simulink library "modVehicle000_cl"  (R2018b)
settings: Solver=VariableStepAuto  StartTime=0.0  StopTime=10.0  RelTol=1e-3
undefined symbols (not defined in the file): constantNormVelBool, constantVelBool, constantVelMag, env, initAngRates, Jinv, m, Minv, MMAddBool, MMOverrideBool, radialMotionBool, sixDoFDynamics, sixDoFDynamics_ul, startControl, vhcl
libraries: vrlib x3, vectorNormalizer_ul x3, eulAng2RotMat_ul x2, dragTurbine_ul x1, fluidDynamicSurface_cl x1, simulink x1, eulDot x1, tethersMoment_cl x1, thrAttachPtKinematics_ul x1
settings Model: Creator=mcobb  LastModifiedBy=mcobb

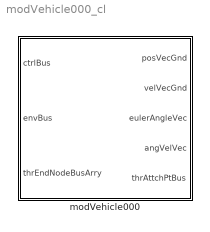
== system modVehicle000_cl ==
  modVehicle000 : Subsystem  VariantControl=VSS_vehicle_vehicle000  mask{vcl=vhcl, rho=env.water.density.Value, grav=env.gravAccel.Value}
      mask prompts: vcl "Vehicle"; rho "Fluid Density"; grav "Gravity"
      mask DialogControl Container9 Prompt: General
      mask DialogControl Container5 Prompt: Vehicle object
      mask DialogControl ParameterGroupVar Prompt: Environmental
      mask Display:
      | image('kite.jpg',[100 100 601 528]/4,'on')
      | 
      | port_label('input',1,'ctrlBus')
      | port_label('input',2,'envBus')
      | port_label('input',3,'thrEndNodeBusArry')
      | 
      | port_label('output',1,'posVecGnd')
      | port_label('output',2,'velVecGnd')
      | port_label('output',3,'eulAng')
      | port_label('output',4,'angVelVec')
      | port_label('output',5,'thrAttchPtBus')

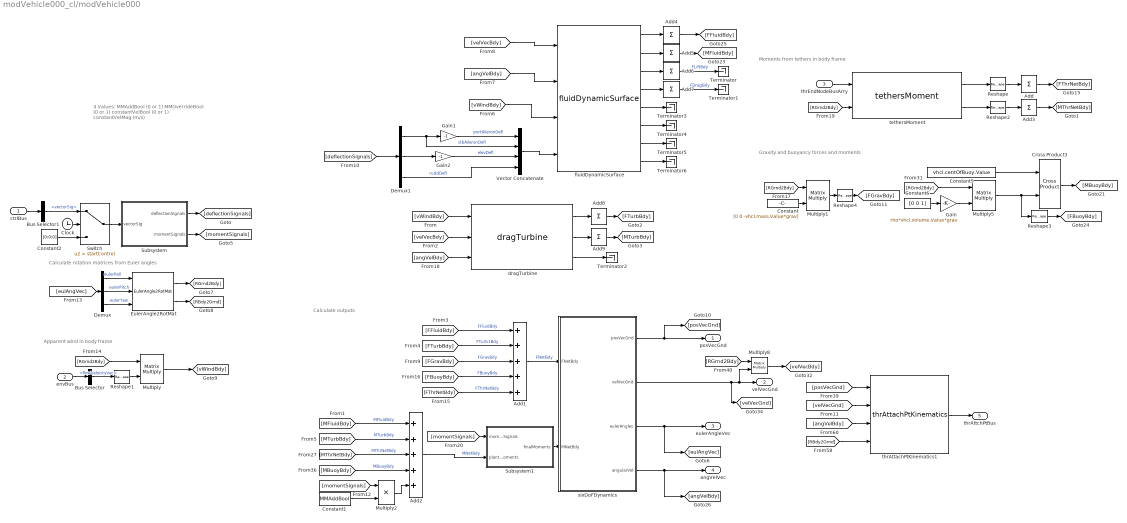
== system modVehicle000_cl/modVehicle000 ==
  note: 4 Values:
      | MMAddBool (0 or 1)
      | MMOverrideBool (0 or 1)
      | constantVelBool (0 or 1)
      | constantVelMag (m/s)
  note: Calculate outputs
  note: Apparent wind in body frame
  note: Calculate rotation matrices from Euler angles
  note: Gravity and buoyancy forces and moments
  note: Moments from tethers in body frame
  ctrlBus : Inport  OutDataTypeStr=Bus: fltCtrlBus
  envBus : Inport  Port=2  OutDataTypeStr=Bus: envBus
  thrEndNodeBusArry : Inport  Port=3
  Add : Sum  Inputs=+  CollapseMode=Specified dimension  CollapseDim=2
  Add1 : Sum  Inputs=+++++
  Add2 : Sum  Inputs=+++++
  Add3 : Sum  Inputs=+  CollapseMode=Specified dimension  CollapseDim=2
  Add{4..9} (6 alike) : Sum  Inputs=1  CollapseMode=Specified dimension  CollapseDim=2
  Bus Selector : BusSelector  OutputSignals=flowVelocityVec
  Bus Selector1 : BusSelector  OutputSignals=vectorSig
  Clock : Clock
  Constant : Constant  Value=[0 0 -vhcl.mass.Value*grav]
  Constant1 : Constant  Value=MMAddBool
  Constant2 : Constant  Value=[0;0;0]
  Constant5 : Constant  Value=vhcl.centOfBuoy.Value
  Constant6 : Constant  Value=[0 0 1]
  Cross Product3 : vrlib/Utilities/Cross Product
      settings: SourceProductBaseCode=VR
  Demux : Demux  Outputs=3
  Demux1 : Demux  Outputs=3
  EulerAngle2RotMat : eulAng2RotMat_ul/EulerAngle2RotMat  SystemSampleTime=-1
  Gain : Gain  Gain=rho*vhcl.volume.Value*grav
  Gain1 : Gain  Gain=-1
  Gain2 : Gain  Gain=-1
  Multiply{,1,5,8} (4 alike) : Product  Multiplication=Matrix(*)
  Multiply2 : Product
  Reshape : Reshape  OutputDimensionality=Customize  OutputDimensions=[3 vhcl.numTethers.Value]
  Reshape1 : Reshape  OutputDimensionality=Column vector (2-D)
  Reshape2 : Reshape  OutputDimensionality=Customize  OutputDimensions=[3 vhcl.numTethers.Value]
  Reshape3 : Reshape  OutputDimensionality=Column vector (2-D)
  Reshape4 : Reshape  OutputDimensionality=Column vector (2-D)
  Subsystem : Subsystem
  Subsystem1 : Subsystem
  Switch : Switch  Criteria=u2 > Threshold  Threshold=startControl
  Terminator{,1..6} (7 alike) : Terminator
  Vector Concatenate : Concatenate  NumInputs=4
  dragTurbine : dragTurbine_ul/dragTurbine  rho_fluid=rho  turb_struct=vhcl.struct('OCT.turb')
  fluidDynamicSurface : fluidDynamicSurface_cl/fluidDynamicSurface  aeroStruct=vcl.struct('OCT.aeroSurf')  fluidDensity=rho
  sixDoFDynamics : Subsystem  AncestorBlock=sixDoFDynamics_ul/sixDoFDynamics  mask{M=vhcl.mass.Value, J=vhcl.inertia.Value, initPos=vhcl.initPosVecGnd.Value, initVel=vhcl.initVelVecGnd.Value, initEulAngs=vhcl.initEulAngBdy.Value, initAngVel=vhcl.initAngVelVecBdy.Value}
      mask prompts: M "Mass"; J "Inertia matrix"; initPos "Initial position"; initVel "Initial velocity"; initEulAngs "Initial Euler Angles"; initAngVel "Initial Angular Velocity Vec"
      mask init:
      | sixDoFDynamics_init
  tethersMoment : tethersMoment_cl/tethersMoment  arms=vhcl.struct('OCT.thrAttch')
  thrAttachPtKinematics1 : thrAttachPtKinematics_ul/thrAttachPtKinematics  atchPts=vhcl.struct('OCT.thrAttch')
  posVecGnd : Outport
  velVecGnd : Outport  Port=2
  eulerAngleVec : Outport  Port=3
  angVelVec : Outport  Port=4
  thrAttchPtBus : Outport  Port=5
  wires:
  Bus Selector/1 -> Reshape1/1  "<flowVelocityVec>"
  [eulAngVec] -> Demux/1
  Demux/2 -> EulerAngle2RotMat/2  "eulerPitch"
  Demux/1 -> EulerAngle2RotMat/1  "eulerRoll"
  Demux/3 -> EulerAngle2RotMat/3  "eulerYaw"
  EulerAngle2RotMat/1 -> [RGrnd2Bdy]
  EulerAngle2RotMat/2 -> [RBdy2Grnd]
  [RGrnd2Bdy] -> Multiply/1
  Multiply/1 -> [vWindBdy]
  [RGrnd2Bdy] -> Multiply1/1
  thrEndNodeBusArry/1 -> tethersMoment/1
  Constant6/1 -> Gain/1
  Multiply5/1 -> Cross Product3/2, Reshape3/1
  [RGrnd2Bdy] -> Multiply5/1
  Cross Product3/1 -> [MBuoyBdy]
  Constant5/1 -> Cross Product3/1
  [MFluidBdy] -> Add2/1  "MFluidBdy"
  [MThrNetBdy] -> Add2/3  "MThrNetBdy"
  [MTurbBdy] -> Add2/2  "MTurbBdy"
  sixDoFDynamics/3(eulerAngles) -> [eulAngVec], eulerAngleVec/1
  sixDoFDynamics/4(angularVel) -> [angVelBdy], angVelVec/1
  [FFluidBdy] -> Add1/1  "FFluidBdy"
  [FTurbBdy] -> Add1/2  "FTurb1Bdy"
  Constant/1 -> Multiply1/2
  fluidDynamicSurface/2 -> Add5/1
  sixDoFDynamics/1(posVecGnd) -> [posVecGnd], posVecGnd/1
  Multiply8/1 -> [velVecBdy]
  [RGrnd2Bdy] -> Multiply8/1
  [angVelBdy] -> thrAttachPtKinematics1/3
  thrAttachPtKinematics1/1 -> thrAttchPtBus/1
  [posVecGnd] -> thrAttachPtKinematics1/1
  [RBdy2Grnd] -> thrAttachPtKinematics1/4
  [velVecGnd] -> thrAttachPtKinematics1/2
  tethersMoment/1 -> Reshape/1
  Reshape/1 -> Add/1
  Add/1 -> [FThrNetBdy]
  [RGrnd2Bdy] -> tethersMoment/2
  Reshape1/1 -> Multiply/2
  Add3/1 -> [MThrNetBdy]
  Reshape2/1 -> Add3/1
  tethersMoment/2 -> Reshape2/1
  Add1/1 -> sixDoFDynamics/1(FNetBdy)  "FNetBdy"
  envBus/1 -> Bus Selector/1
  fluidDynamicSurface/1 -> Add4/1
  fluidDynamicSurface/3 -> Add6/1
  fluidDynamicSurface/4 -> Add7/1
  [vWindBdy] -> fluidDynamicSurface/3
  [angVelBdy] -> fluidDynamicSurface/2
  [velVecBdy] -> fluidDynamicSurface/1
  Add4/1 -> [FFluidBdy]
  Add5/1 -> [MFluidBdy]
  Add6/1 -> Terminator/1  "FLiftBdy"
  Add7/1 -> Terminator1/1  "FDragBdy"
  dragTurbine/1 -> Add8/1
  dragTurbine/2 -> Add9/1
  Add8/1 -> [FTurbBdy]
  Add9/1 -> [MTurbBdy]
  dragTurbine/3 -> Terminator2/1
  [vWindBdy] -> dragTurbine/1
  [velVecBdy] -> dragTurbine/2
  [angVelBdy] -> dragTurbine/3
  [MBuoyBdy] -> Add2/4  "MBuoyBdy"
  [FThrNetBdy] -> Add1/5  "FThrNetBdy"
  [FBuoyBdy] -> Add1/4  "FBuoyBdy"
  [FGravBdy] -> Add1/3  "FGravBdy"
  Gain/1 -> Multiply5/2
  Vector Concatenate/1 -> fluidDynamicSurface/4
  ctrlBus/1 -> Bus Selector1/1
  [deflectionSignals] -> Demux1/1
  Demux1/3 -> Vector Concatenate/4  "ruddDefl"
  Demux1/2 -> Gain2/1
  Gain1/1 -> Vector Concatenate/1  "portAileronDefl"
  Demux1/1 -> Vector Concatenate/2, Gain1/1  "stbAileronDefl"
  Gain2/1 -> Vector Concatenate/3  "elevDefl"
  Subsystem/1(deflectionSignals) -> [deflectionSignals]
  Subsystem1/1(finalMoments) -> sixDoFDynamics/2(MNetBdy)
  Add2/1 -> Subsystem1/2("plantCreatedMoments ")  "MNetBdy"
  [momentSignals] -> Subsystem1/1(momentSignals)
  sixDoFDynamics/2(velVecGnd) -> velVecGnd/1, Multiply8/2, [velVecGnd]
  [momentSignals] -> Multiply2/1
  Multiply2/1 -> Add2/5
  Constant1/1 -> Multiply2/2
  fluidDynamicSurface/5 -> Terminator3/1
  fluidDynamicSurface/7 -> Terminator5/1
  fluidDynamicSurface/6 -> Terminator4/1
  Reshape3/1 -> [FBuoyBdy]
  Multiply1/1 -> Reshape4/1
  Reshape4/1 -> [FGravBdy]
  Subsystem/2(momentSignals) -> [momentSignals]
  fluidDynamicSurface/8 -> Terminator6/1
  Clock/1 -> Switch/2
  Constant2/1 -> Switch/3
  Bus Selector1/1 -> Switch/1  "<vectorSig>"
  Switch/1 -> Subsystem/1(vectorSig)

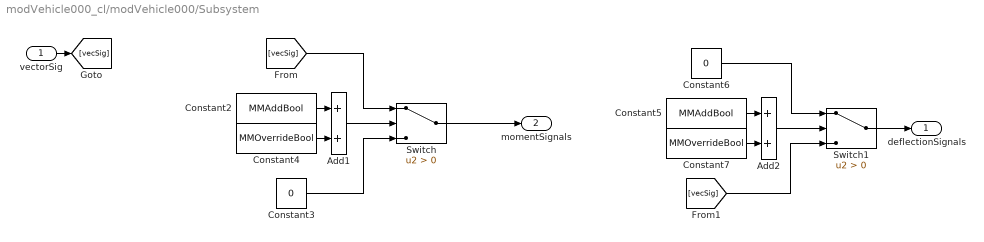
== system modVehicle000_cl/modVehicle000/Subsystem ==
  vectorSig : Inport
  Add1 : Sum
  Add2 : Sum
  Constant2 : Constant  Value=MMAddBool
  Constant3 : Constant  Value=0
  Constant4 : Constant  Value=MMOverrideBool
  Constant5 : Constant  Value=MMAddBool
  Constant6 : Constant  Value=0
  Constant7 : Constant  Value=MMOverrideBool
  Switch : Switch  Criteria=u2 > Threshold
  Switch1 : Switch  Criteria=u2 > Threshold
  deflectionSignals : Outport
  momentSignals : Outport  Port=2
  wires:
  Constant3/1 -> Switch/3
  [vecSig] -> Switch/1
  Add1/1 -> Switch/2
  Constant2/1 -> Add1/1
  Constant4/1 -> Add1/2
  Switch/1 -> momentSignals/1
  [vecSig] -> Switch1/3
  Constant7/1 -> Add2/2
  Constant5/1 -> Add2/1
  Add2/1 -> Switch1/2
  Switch1/1 -> deflectionSignals/1
  vectorSig/1 -> [vecSig]
  Constant6/1 -> Switch1/1

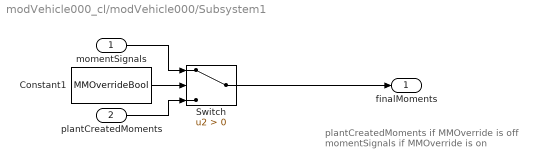
== system modVehicle000_cl/modVehicle000/Subsystem1 ==
  note: plantCreatedMoments if MMOverride is off
      | momentSignals if MMOverride is on
  momentSignals : Inport
  "plantCreatedMoments " : Inport  Port=2
  Constant1 : Constant  Value=MMOverrideBool
  Switch : Switch  Criteria=u2 > Threshold
  finalMoments : Outport
  wires:
  Constant1/1 -> Switch/2
  momentSignals/1 -> Switch/1
  "plantCreatedMoments "/1 -> Switch/3
  Switch/1 -> finalMoments/1

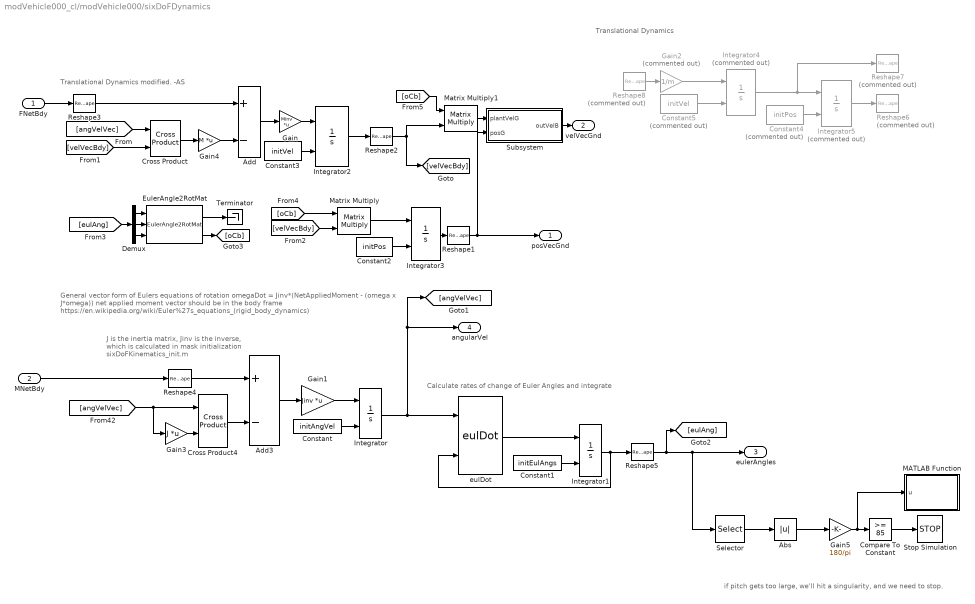
== system modVehicle000_cl/modVehicle000/sixDoFDynamics ==
  note: Translational Dynamics
  note: J is the inertia matrix, Jinv is the inverse,
      | which is calculated in mask initialization
      | sixDoFKinematics_init.m
  note: General vector form of Eulers equations of rotation
      | omegaDot = Jinv*(NetAppliedMoment - (omega x J*omega))
      | net applied moment vector should be in the body frame
      | https://en.wikipedia.org/wiki/Euler%27s_equations_(rigid_body_dynamics)
  note: Calculate rates of change of Euler Angles and integrate
  note: Translational Dynamics modified. -AS
  note: if pitch gets too large, we'll hit a singularity, and we need to stop.
  FNetBdy : Inport
  MNetBdy : Inport  Port=2
  Abs : Abs
  Add : Sum  Inputs=+-
  Add3 : Sum  Inputs=+-
  Compare To Constant : simulink/Logic and Bit Operations/Compare To Constant  relop=>=  const=85  OutDataTypeStr=boolean
  Constant : Constant  Value=initAngVel
  Constant1 : Constant  Value=initEulAngs
  Constant2 : Constant  Value=initPos
  Constant3 : Constant  Value=initVel
  Constant4 : Constant  Commented=on  Value=initPos
  Constant5 : Constant  Commented=on  Value=initVel
  Cross Product : vrlib/Utilities/Cross Product
      settings: SourceProductBaseCode=VR
  Cross Product4 : vrlib/Utilities/Cross Product
      settings: SourceProductBaseCode=VR
  Demux : Demux  Outputs=3
  EulerAngle2RotMat : eulAng2RotMat_ul/EulerAngle2RotMat  SystemSampleTime=-1
  Gain : Gain  Gain=Minv  Multiplication=Matrix(K*u)
  Gain1 : Gain  Gain=Jinv  Multiplication=Matrix(K*u)
  Gain2 : Gain  Commented=on  Gain=1/m
  Gain3 : Gain  Gain=J  Multiplication=Matrix(K*u)
  Gain4 : Gain  Gain=M  Multiplication=Matrix(K*u)
  Gain5 : Gain  Gain=180/pi
  Integrator : Integrator  InitialConditionSource=external  InitialCondition=initAngRates
  Integrator1 : Integrator  InitialConditionSource=external  InitialCondition=initEulAngs
  Integrator2 : Integrator  InitialConditionSource=external  InitialCondition=initVel
  Integrator3 : Integrator  InitialConditionSource=external  InitialCondition=initPos
  Integrator4 : Integrator  Commented=on  InitialConditionSource=external  InitialCondition=initVel
  Integrator5 : Integrator  Commented=on  InitialConditionSource=external  InitialCondition=initPos
  MATLAB Function : MATLAB Function  TreatAsAtomicUnit=on
  Matrix Multiply : Product  Multiplication=Matrix(*)
  Matrix Multiply1 : Product  Multiplication=Matrix(*)
  Reshape{1..5} (5 alike) : Reshape  OutputDimensionality=Column vector (2-D)
  Reshape6 : Reshape  Commented=on  OutputDimensionality=Column vector (2-D)
  Reshape7 : Reshape  Commented=on  OutputDimensionality=Column vector (2-D)
  Reshape8 : Reshape  Commented=on  OutputDimensionality=Column vector (2-D)
  Selector : Selector  InputPortWidth=3  IndexOptions=Index vector (dialog)  Indices=2  OutputSizes=1
  Stop Simulation : Stop
  Subsystem : Subsystem
  Terminator : Terminator
  eulDot : eulDot/eulDot  SystemSampleTime=-1
  posVecGnd : Outport
  velVecGnd : Outport  Port=2
  eulerAngles : Outport  Port=3
  angularVel : Outport  Port=4
  wires:
  Gain5/1 -> MATLAB Function/1(u), Compare To Constant/1
  Abs/1 -> Gain5/1
  Selector/1 -> Abs/1
  [oCb] -> Matrix Multiply1/1
  [oCb] -> Matrix Multiply/1
  EulerAngle2RotMat/2 -> [oCb]
  EulerAngle2RotMat/1 -> Terminator/1
  Reshape1/1 -> posVecGnd/1, Subsystem/2(posG)
  Matrix Multiply/1 -> Integrator3/1
  [velVecBdy] -> Matrix Multiply/2
  Demux/3 -> EulerAngle2RotMat/3
  Demux/2 -> EulerAngle2RotMat/2
  Demux/1 -> EulerAngle2RotMat/1
  [eulAng] -> Demux/1
  Integrator2/1 -> Reshape2/1
  [velVecBdy] -> Cross Product/2
  [angVelVec] -> Cross Product/1
  Gain/1 -> Integrator2/1
  Add/1 -> Gain/1
  Gain4/1 -> Add/2
  Reshape3/1 -> Add/1
  Cross Product/1 -> Gain4/1
  Reshape8/1 -> Gain2/1
  Gain2/1 -> Integrator4/1
  Integrator4/1 -> Integrator5/1, Reshape7/1
  Constant5/1 -> Integrator4/2
  Integrator5/1 -> Reshape6/1
  Constant4/1 -> Integrator5/2
  Reshape5/1 -> eulerAngles/1, Selector/1, [eulAng]
  Reshape4/1 -> Add3/1
  Constant3/1 -> Integrator2/2
  Constant2/1 -> Integrator3/2
  Constant1/1 -> Integrator1/2
  eulDot/1 -> Integrator1/1
  Constant/1 -> Integrator/2
  Integrator3/1 -> Reshape1/1
  FNetBdy/1 -> Reshape3/1
  Cross Product4/1 -> Add3/2
  Gain1/1 -> Integrator/1
  Integrator1/1 -> Reshape5/1, eulDot/2
  Add3/1 -> Gain1/1
  Integrator/1 -> [angVelVec], angularVel/1, eulDot/1
  Gain3/1 -> Cross Product4/2
  [angVelVec] -> Gain3/1, Cross Product4/1
  MNetBdy/1 -> Reshape4/1
  Reshape2/1 -> [velVecBdy], Matrix Multiply1/2
  Compare To Constant/1 -> Stop Simulation/1
  Matrix Multiply1/1 -> Subsystem/1(plantVelG)
  Subsystem/1("outVelB ") -> velVecGnd/1

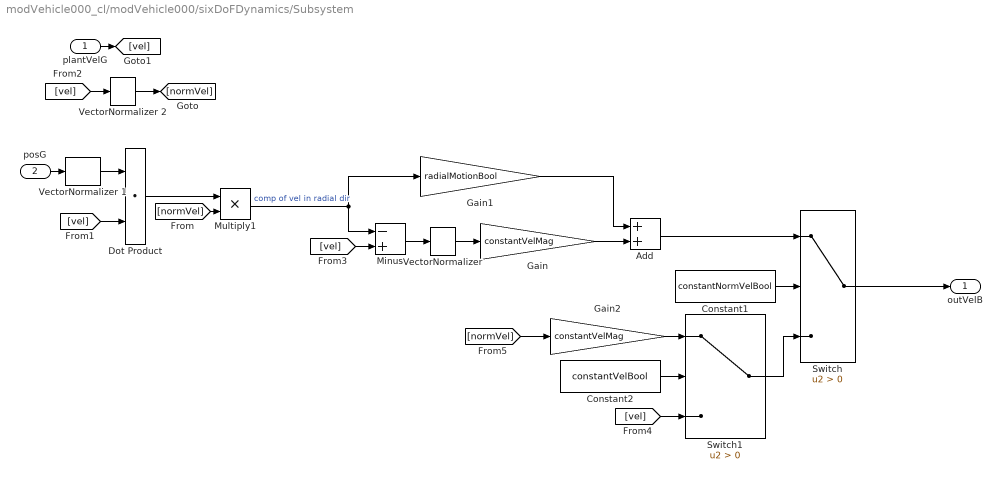
== system modVehicle000_cl/modVehicle000/sixDoFDynamics/Subsystem ==
  plantVelG : Inport
  posG : Inport  Port=2
  Add : Sum
  Constant1 : Constant  Value=constantNormVelBool  VectorParams1D=off
  Constant2 : Constant  Value=constantVelBool  VectorParams1D=off
  Dot Product : DotProduct  InputSameDT=on  OutDataTypeStr=Inherit: Inherit via internal rule
  Gain : Gain  Gain=constantVelMag
  Gain1 : Gain  Gain=radialMotionBool
  Gain2 : Gain  Gain=constantVelMag
  Minus : Sum  Inputs=-+
  Multiply1 : Product
  Switch : Switch  Criteria=u2 > Threshold
  Switch1 : Switch  Criteria=u2 > Threshold
  "VectorNormalizer " : vectorNormalizer_ul/VectorNormalizer   SystemSampleTime=-1
  VectorNormalizer 1 : vectorNormalizer_ul/VectorNormalizer   SystemSampleTime=-1
  VectorNormalizer 2 : vectorNormalizer_ul/VectorNormalizer   SystemSampleTime=-1
  "outVelB " : Outport
  wires:
  Add/1 -> Switch/1
  Switch/1 -> "outVelB "/1
  Constant1/1 -> Switch/2
  "VectorNormalizer "/1 -> Gain/1
  posG/1 -> VectorNormalizer 1/1
  VectorNormalizer 1/1 -> Dot Product/1
  Minus/1 -> "VectorNormalizer "/1
  Gain/1 -> Add/2
  Multiply1/1 -> Minus/1, Gain1/1  "comp of vel in radial dir"
  Gain1/1 -> Add/1
  VectorNormalizer 2/1 -> [normVel]
  Dot Product/1 -> Multiply1/1
  [normVel] -> Multiply1/2
  plantVelG/1 -> [vel]
  [vel] -> Dot Product/2
  [vel] -> VectorNormalizer 2/1
  [vel] -> Minus/2
  Switch1/1 -> Switch/3
  [vel] -> Switch1/3
  Constant2/1 -> Switch1/2
  [normVel] -> Gain2/1
  Gain2/1 -> Switch1/1

== matlab function modVehicle000_cl/modVehicle000/sixDoFDynamics/MATLAB Function ==
  data: u input
function fcn(u)
    if u>85
        fprintf("Executed Stop because pitch = %4.2f\n",u)
    end
end
